simulink model "System"  (R2023a)
settings: Solver=VariableStepAuto  StartTime=0.0  StopTime=10.0  RelTol=1e-3
model workspace (MAT data in the model file):
  T = Simulink.Parameter
  T.DataType = 'auto'
  T.Complexity = 'real'
  T.Dimensions = [1 1]
settings Model: Creator=Francesca  LastModifiedBy=Francesca

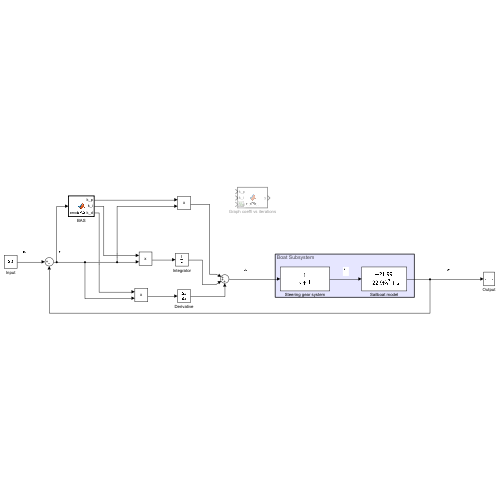
[thumbnail: Simulink's stored preview of the top-level diagram]
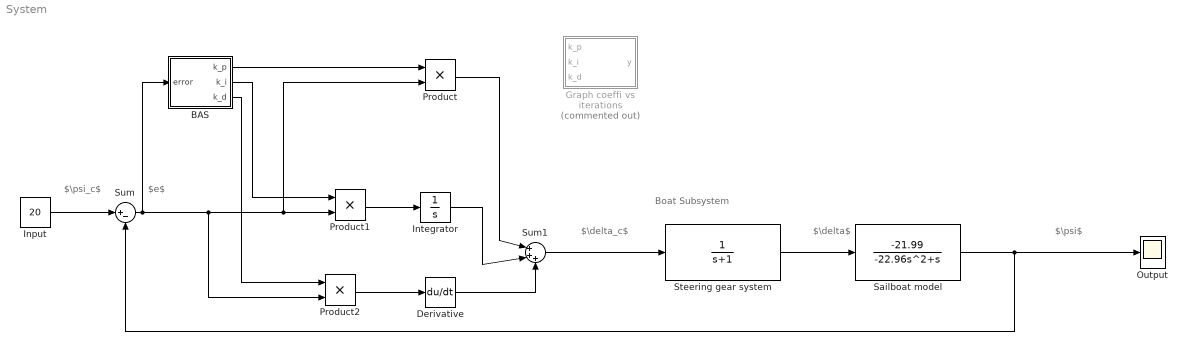
== system System ==
  note: Boat Subsystem
  note: $\psi_c$
  note: $\psi$
  note: $\delta_c$
  note: $e$
  note: $\delta$
  BAS : MATLAB Function  TreatAsAtomicUnit=on
  Derivative : Derivative
  Graph coeffi vs iterations : MATLAB Function  Commented=on  TreatAsAtomicUnit=on
  Input : Constant  Value=20
  Integrator : Integrator
  Output : Scope
  Product : Product
  Product1 : Product
  Product2 : Product
  Sailboat model : TransferFcn  Numerator=[-21.99]  Denominator=[-22.96 1 0]
  Steering gear system : TransferFcn  Denominator=[1 1]
  Sum : Sum  Inputs=|+-
  Sum1 : Sum  Inputs=|+++
  wires:
  Input/1 -> Sum/1
  Sailboat model/1 -> Sum/2, Output/1
  Steering gear system/1 -> Sailboat model/1
  Sum/1 -> Product1/2, Product/2, Product2/2, BAS/1(error)
  Sum1/1 -> Steering gear system/1
  Integrator/1 -> Sum1/2
  Derivative/1 -> Sum1/3
  BAS/1(k_p) -> Product/1
  Product/1 -> Sum1/1
  Product1/1 -> Integrator/1
  BAS/2(k_i) -> Product1/1
  Product2/1 -> Derivative/1
  BAS/3(k_d) -> Product2/1

== matlab function System/BAS ==
  data: error input; k_p output; k_i output; k_d output
% function y = fcn(u)
% 
% y = u;
function [k_p, k_i, k_d] = BAS(error)

n_dims = 3;     % search space dimension
d = 3;          % antennae's sensing length
% d0 = 0.001;     % Constant
eta = 0.95;     % step factor
delta = 10;     % search step size
n = 100;        % max number of iterations

sz = [n_dims, 1];
x = rand(sz);       % random position of beetle
x = x / norm(x);

% Data history for visualization
x_history = zeros(sz) * ones(1, n);
y_history = zeros(n, 1);

% First cost function value
x_best = x;
y_best = cost_fun(x);
y_best_history = zeros(n,1);

% Iterations
for i=1:n
    % Data history for visualization
    y_best_history(i) = y_best;
    y = cost_fun(x);        % evaluate cost function in current position
    x_history(:, i) = x;    
    y_history(i) = y;

    % Random search direction
    b = rand(sz);      
    b = b / norm(b);

    % Left and right antennae's position update
    x_r = x + d * b;    
    x_l = x - d * b;

    % Update beetle's position
    x = x + delta * sign(cost_fun(x_l) - cost_fun(x_r)) * b;
    y = cost_fun(x);

    if  y < y_best
        y_best = y;
        x_best = x;
        k_p = x_best(1);
        k_i = x_best(2);
        k_d = x_best(3);
    end
    
    % Update d and delta
    % Comment next two lines to set d and delta as constants
    % d = d * eta + d0;
    delta = delta * eta;
    
end
end

== matlab function System/Graph coeffi vs iterations ==
  data: k_p input; y output; k_i input; k_d input
function y = doPlot(k_p,k_i, k_d)

end
